simulink subsystem "DataMemoryMUX"  (R2024b)
settings: Solver=VariableStepAuto  StartTime=0.0  StopTime=10.0  RelTol=1e-3
settings Model: Creator=stefano  LastModifiedBy=stefano

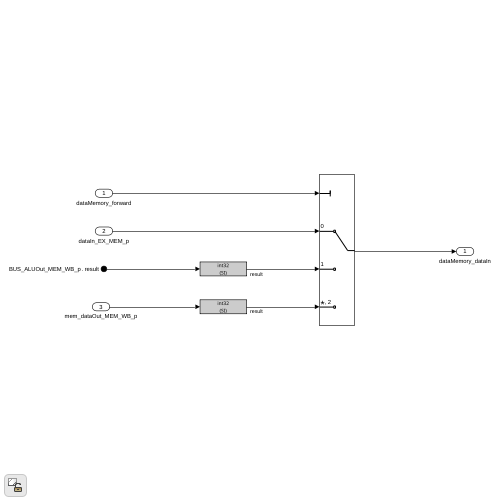
[thumbnail: Simulink's stored preview of the top-level diagram]
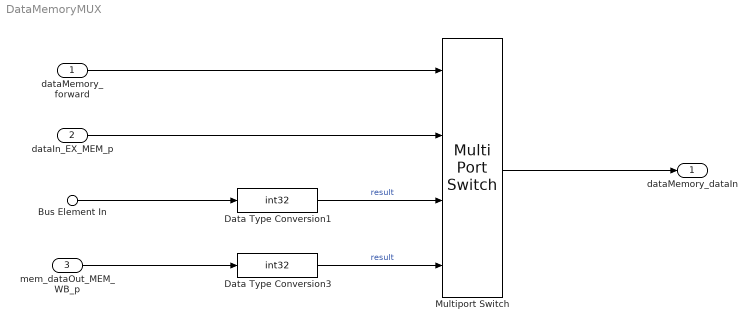
== system DataMemoryMUX ==
  dataMemory_forward : Inport
  dataIn_EX_MEM_p : Inport  Port=2
  mem_dataOut_MEM_WB_p : Inport  Port=3
  Bus Element In : Inport  Port=4  PortName=BUS_ALUOut_MEM_WB_p  Element=result
  Data Type Conversion1 : DataTypeConversion  OutDataTypeStr=int32  ConvertRealWorld=Stored Integer (SI)  SaturateOnIntegerOverflow=off  RndMeth=Floor
  Data Type Conversion3 : DataTypeConversion  OutDataTypeStr=int32  ConvertRealWorld=Stored Integer (SI)  SaturateOnIntegerOverflow=off  RndMeth=Floor
  Multiport Switch : MultiPortSwitch  DataPortOrder=Zero-based contiguous  zeroidx=on  SaturateOnIntegerOverflow=off  InputSameDT=off
  dataMemory_dataIn : Outport
  wires:
  dataIn_EX_MEM_p/1 -> Multiport Switch/2
  dataMemory_forward/1 -> Multiport Switch/1
  mem_dataOut_MEM_WB_p/1 -> Data Type Conversion3/1
  Data Type Conversion3/1 -> Multiport Switch/4  "result"
  Data Type Conversion1/1 -> Multiport Switch/3  "result"
  Multiport Switch/1 -> dataMemory_dataIn/1
  Bus Element In/1 -> Data Type Conversion1/1
